simulink model "sensor_array_test"  (R2020a)
settings: Solver=VariableStepAuto  StartTime=0.0  StopTime=0.5  RelTol=1e-3
undefined symbols (not defined in the file or in its folder): duration, effort, index, joint_name, left_front, left_rear, model_name, right_front, right_rear, robotracer
libraries: robotgazebolib x24, simulink x3
settings Model: Creator=under  LastModifiedBy=under

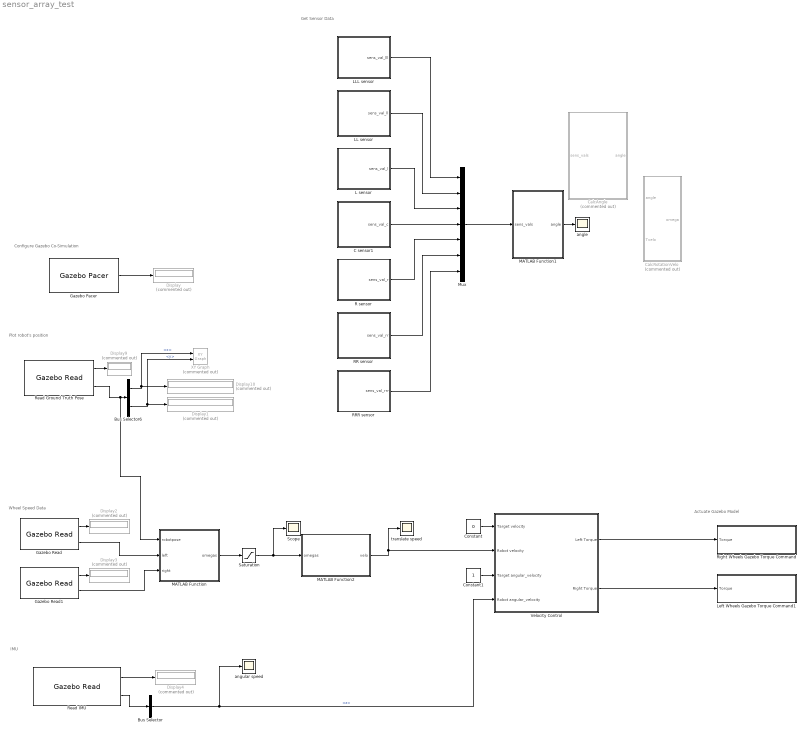
== system sensor_array_test ==
  note: Configure Gazebo Co-Simulation
  note: Plot robot's position
  note: Wheel Speed Data
  note: Actuate Gazebo Model
  note: IMU
  note: Get Sensor Data
  Bus Selector : BusSelector  OutputSignals=angular_velocity.z
  Bus Selector6 : BusSelector  OutputSignals=position.x,position.y
  C sensor1 : Subsystem
  CalcAngle : MATLAB Function  Commented=on  TreatAsAtomicUnit=on
  CalcRotationVelo : MATLAB Function  Commented=on  TreatAsAtomicUnit=on
  Constant : Constant  Value=0
  Constant1 : Constant
  Display{,1..4,9..10} (7 alike) : Display  Commented=on
  Gazebo Pacer : robotgazebolib/Gazebo Pacer  ResetBehavior=Reset Gazebo simulation time and scene  SampleTime=0.001
      settings: SourceProductBaseCode=RO
  Gazebo Read : robotgazebolib/Gazebo Read  topicSource=From Gazebo  topic=/gazebo/ground_truth/world_pose/robotracer/left_front_wheel  messageType=gazebo_msgs/Pose  sampleTime=0.001
      settings: SourceProductBaseCode=RO
  Gazebo Read1 : robotgazebolib/Gazebo Read  topicSource=From Gazebo  topic=/gazebo/ground_truth/world_pose/robotracer/right_front_wheel  messageType=gazebo_msgs/Pose  sampleTime=0.001
      settings: SourceProductBaseCode=RO
  L sensor : Subsystem
  LL sensor : Subsystem
  LLL sensor : Subsystem
  Left Wheels Gazebo Torque Command1 : Subsystem
  MATLAB Function : MATLAB Function  TreatAsAtomicUnit=on
  MATLAB Function1 : MATLAB Function  TreatAsAtomicUnit=on
  MATLAB Function2 : MATLAB Function  TreatAsAtomicUnit=on
  Mux : Mux  Inputs=7
  R sensor : Subsystem
  RR sensor : Subsystem
  RRR sensor : Subsystem
  Read Ground Truth Pose : robotgazebolib/Gazebo Read  topicSource=From Gazebo  topic=/gazebo/ground_truth/world_pose/robotracer/chassis  messageType=gazebo_msgs/Pose  sampleTime=0.001
      settings: SourceProductBaseCode=RO
  Read IMU : robotgazebolib/Gazebo Read  topicSource=From Gazebo  topic=/gazebo/default/robotracer/chassis/imu/imu  messageType=gazebo_msgs/IMU  sampleTime=0.01
      settings: SourceProductBaseCode=RO
  Right Wheels Gazebo Torque Command : Subsystem
  Saturation : Saturate  UpperLimit=90  LowerLimit=-90
  Scope : Scope
  Velocity Control : Subsystem
  XY Graph : simulink/Sinks/XY Graph  Commented=on  xmin=-1  xmax=1  ymin=-1  ymax=1  st=-1
  angle : Scope
  angular speed : Scope
  translate speed : Scope
  wires:
  Gazebo Pacer/1 -> Display/1
  Bus Selector6/1 -> XY Graph/1, Display10/1  "<x>"
  Bus Selector6/2 -> XY Graph/2, Display1/1  "<y>"
  MATLAB Function/1(omegas) -> Saturation/1
  Read Ground Truth Pose/2 -> MATLAB Function/1(robotpose), Bus Selector6/1
  Gazebo Read1/2 -> MATLAB Function/3(right)
  Gazebo Read/2 -> MATLAB Function/2(left)
  Gazebo Read1/1 -> Display3/1
  Gazebo Read/1 -> Display2/1
  Read Ground Truth Pose/1 -> Display9/1
  Saturation/1 -> MATLAB Function2/1(omegas), Scope/1
  MATLAB Function2/1(velo) -> Velocity Control/2(Robot velocity), translate speed/1
  Constant/1 -> Velocity Control/1(Target velocity)
  Read IMU/2 -> Bus Selector/1
  Read IMU/1 -> Display4/1
  Bus Selector/1 -> Velocity Control/4(Robot angular_velocity), angular speed/1  "<z>"
  Constant1/1 -> Velocity Control/3(Target angular_velocity)
  Velocity Control/1(Left Torque) -> Right Wheels Gazebo Torque Command/1(Torque)
  Velocity Control/2(Right Torque) -> Left Wheels Gazebo Torque Command1/1(Torque)
  C sensor1/1(sens_val_c) -> Mux/4
  L sensor/1(sens_val_l) -> Mux/3
  LL sensor/1(sens_val_ll) -> Mux/2
  LLL sensor/1(sens_val_lll) -> Mux/1
  R sensor/1(sens_val_r) -> Mux/5
  RR sensor/1(sens_val_rr) -> Mux/6
  RRR sensor/1(sens_val_rrr) -> Mux/7
  Mux/1 -> MATLAB Function1/1(sens_vals)
  MATLAB Function1/1(angle) -> angle/1

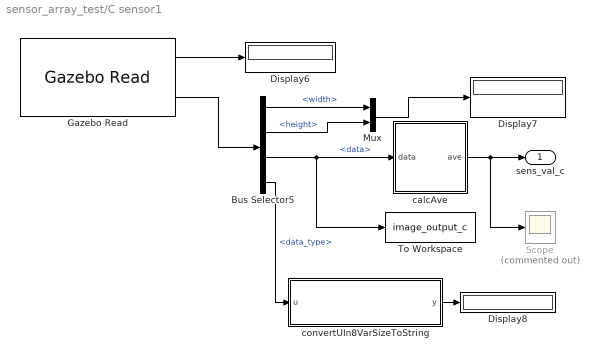
== system sensor_array_test/C sensor1 ==
  Bus Selector5 : BusSelector  OutputSignals=width,height,data,data_type
  Display6 : Display
  Display7 : Display
  Display8 : Display
  Gazebo Read : robotgazebolib/Gazebo Read  topicSource=From Gazebo  topic=/gazebo/default/robotracer/camera_link/camera_c/image  messageType=gazebo_msgs/Image  sampleTime=0.01
      settings: SourceProductBaseCode=RO
  Mux : Mux  Inputs=2
  Scope : Scope  Commented=on
  To Workspace : ToWorkspace  VariableName=image_output_c  SaveFormat=Structure With Time  SampleTime=-1
  calcAve : MATLAB Function  TreatAsAtomicUnit=on
  convertUIn8VarSizeToString : MATLAB Function  TreatAsAtomicUnit=on
  sens_val_c : Outport
  wires:
  calcAve/1(ave) -> sens_val_c/1, Scope/1
  Mux/1 -> Display7/1
  convertUIn8VarSizeToString/1(y) -> Display8/1
  Bus Selector5/2 -> Mux/2  "<height>"
  Bus Selector5/3 -> calcAve/1(data), To Workspace/1  "<data>"
  Bus Selector5/4 -> convertUIn8VarSizeToString/1(u)  "<data_type>"
  Gazebo Read/1 -> Display6/1
  Bus Selector5/1 -> Mux/1  "<width>"
  Gazebo Read/2 -> Bus Selector5/1

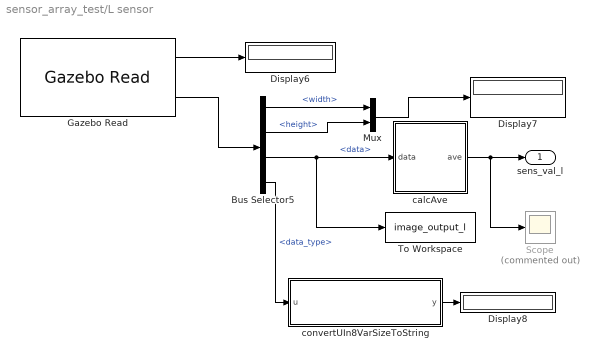
== system sensor_array_test/L sensor ==
  Bus Selector5 : BusSelector  OutputSignals=width,height,data,data_type
  Display6 : Display
  Display7 : Display
  Display8 : Display
  Gazebo Read : robotgazebolib/Gazebo Read  topicSource=From Gazebo  topic=/gazebo/default/robotracer/camera_link/camera_l/image  messageType=gazebo_msgs/Image  sampleTime=0.01
      settings: SourceProductBaseCode=RO
  Mux : Mux  Inputs=2
  Scope : Scope  Commented=on
  To Workspace : ToWorkspace  VariableName=image_output_l  SaveFormat=Structure With Time  SampleTime=-1
  calcAve : MATLAB Function  TreatAsAtomicUnit=on
  convertUIn8VarSizeToString : MATLAB Function  TreatAsAtomicUnit=on
  sens_val_l : Outport
  wires:
  calcAve/1(ave) -> sens_val_l/1, Scope/1
  Mux/1 -> Display7/1
  convertUIn8VarSizeToString/1(y) -> Display8/1
  Bus Selector5/2 -> Mux/2  "<height>"
  Bus Selector5/3 -> calcAve/1(data), To Workspace/1  "<data>"
  Bus Selector5/4 -> convertUIn8VarSizeToString/1(u)  "<data_type>"
  Gazebo Read/1 -> Display6/1
  Bus Selector5/1 -> Mux/1  "<width>"
  Gazebo Read/2 -> Bus Selector5/1

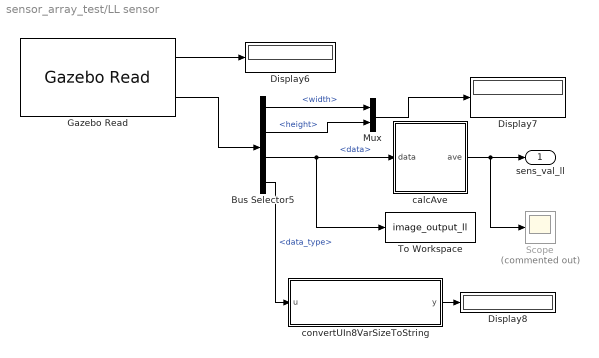
== system sensor_array_test/LL sensor ==
  Bus Selector5 : BusSelector  OutputSignals=width,height,data,data_type
  Display6 : Display
  Display7 : Display
  Display8 : Display
  Gazebo Read : robotgazebolib/Gazebo Read  topicSource=From Gazebo  topic=/gazebo/default/robotracer/camera_link/camera_ll/image  messageType=gazebo_msgs/Image  sampleTime=0.01
      settings: SourceProductBaseCode=RO
  Mux : Mux  Inputs=2
  Scope : Scope  Commented=on
  To Workspace : ToWorkspace  VariableName=image_output_ll  SaveFormat=Structure With Time  SampleTime=-1
  calcAve : MATLAB Function  TreatAsAtomicUnit=on
  convertUIn8VarSizeToString : MATLAB Function  TreatAsAtomicUnit=on
  sens_val_ll : Outport
  wires:
  calcAve/1(ave) -> sens_val_ll/1, Scope/1
  Mux/1 -> Display7/1
  convertUIn8VarSizeToString/1(y) -> Display8/1
  Bus Selector5/2 -> Mux/2  "<height>"
  Bus Selector5/3 -> calcAve/1(data), To Workspace/1  "<data>"
  Bus Selector5/4 -> convertUIn8VarSizeToString/1(u)  "<data_type>"
  Gazebo Read/1 -> Display6/1
  Bus Selector5/1 -> Mux/1  "<width>"
  Gazebo Read/2 -> Bus Selector5/1

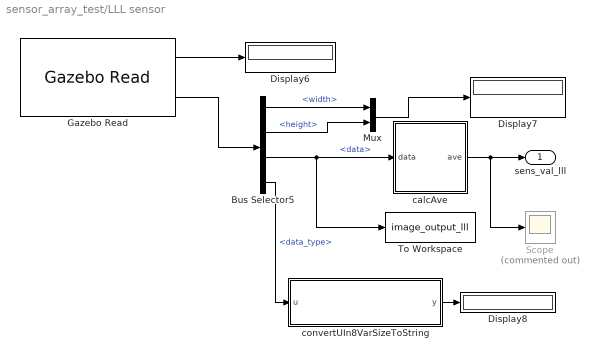
== system sensor_array_test/LLL sensor ==
  Bus Selector5 : BusSelector  OutputSignals=width,height,data,data_type
  Display6 : Display
  Display7 : Display
  Display8 : Display
  Gazebo Read : robotgazebolib/Gazebo Read  topicSource=From Gazebo  topic=/gazebo/default/robotracer/camera_link/camera_lll/image  messageType=gazebo_msgs/Image  sampleTime=0.01
      settings: SourceProductBaseCode=RO
  Mux : Mux  Inputs=2
  Scope : Scope  Commented=on
  To Workspace : ToWorkspace  VariableName=image_output_lll  SaveFormat=Structure With Time  SampleTime=-1
  calcAve : MATLAB Function  TreatAsAtomicUnit=on
  convertUIn8VarSizeToString : MATLAB Function  TreatAsAtomicUnit=on
  sens_val_lll : Outport
  wires:
  calcAve/1(ave) -> sens_val_lll/1, Scope/1
  Mux/1 -> Display7/1
  convertUIn8VarSizeToString/1(y) -> Display8/1
  Bus Selector5/2 -> Mux/2  "<height>"
  Bus Selector5/3 -> calcAve/1(data), To Workspace/1  "<data>"
  Bus Selector5/4 -> convertUIn8VarSizeToString/1(u)  "<data_type>"
  Gazebo Read/1 -> Display6/1
  Bus Selector5/1 -> Mux/1  "<width>"
  Gazebo Read/2 -> Bus Selector5/1

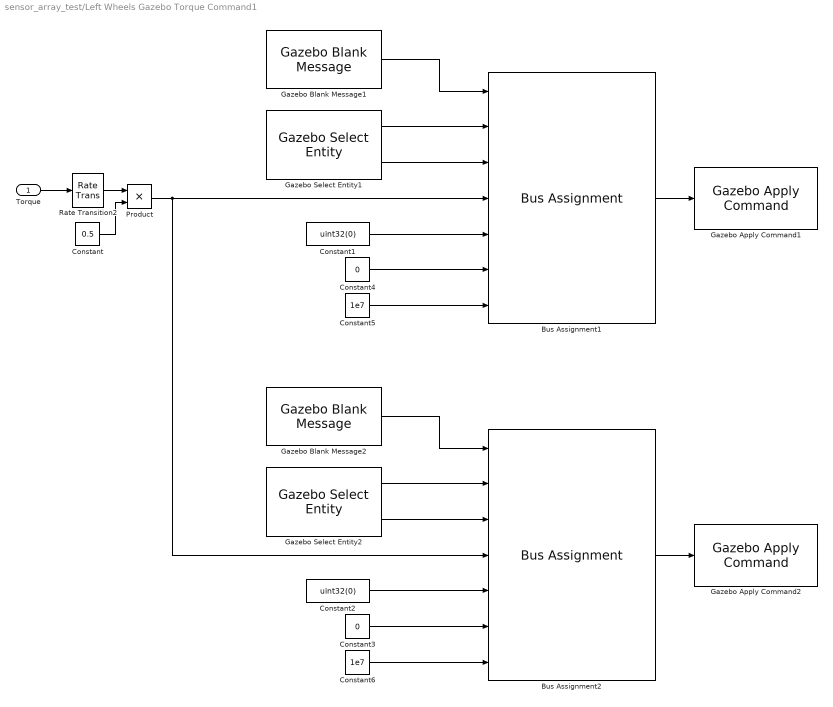
== system sensor_array_test/Left Wheels Gazebo Torque Command1 ==
  Torque : Inport
  Bus Assignment1 : BusAssignment  AssignedSignals=model_name,joint_name,effort,index,duration.seconds,duration.nano_seconds
  Bus Assignment2 : BusAssignment  AssignedSignals=model_name,joint_name,effort,index,duration.seconds,duration.nano_seconds
  Constant : Constant  Value=0.5
  Constant1 : Constant  Value=uint32(0)
  Constant2 : Constant  Value=uint32(0)
  Constant3 : Constant  Value=0
  Constant4 : Constant  Value=0
  Constant5 : Constant  Value=1e7
  Constant6 : Constant  Value=1e7
  Gazebo Apply Command1 : robotgazebolib/Gazebo Apply Command  cmdType=ApplyJointTorque  sampleTime=0.01
      settings: SourceProductBaseCode=RO
  Gazebo Apply Command2 : robotgazebolib/Gazebo Apply Command  cmdType=ApplyJointTorque  sampleTime=0.01
      settings: SourceProductBaseCode=RO
  Gazebo Blank Message1 : robotgazebolib/Gazebo Blank Message  msgType=ApplyJointTorque  sampleTime=0.01  busName='Gazebo_SL_Bus_gazebo_msgs_ApplyJointTorque'
      settings: SourceProductBaseCode=RO
  Gazebo Blank Message2 : robotgazebolib/Gazebo Blank Message  msgType=ApplyJointTorque  sampleTime=0.01  busName='Gazebo_SL_Bus_gazebo_msgs_ApplyJointTorque'
      settings: SourceProductBaseCode=RO
  Gazebo Select Entity1 : robotgazebolib/Gazebo Select Entity  modelElemName=robotracer/left_front  outputArraySize=128  OutputLabel=Joint  SelectType=Joint
      settings: SourceProductBaseCode=RO
  Gazebo Select Entity2 : robotgazebolib/Gazebo Select Entity  modelElemName=robotracer/left_rear  outputArraySize=128  OutputLabel=Joint  SelectType=Joint
      settings: SourceProductBaseCode=RO
  Product : Product
  Rate Transition2 : RateTransition
  wires:
  Bus Assignment1/1 -> Gazebo Apply Command1/1
  Constant5/1 -> Bus Assignment1/7
  Gazebo Blank Message1/1 -> Bus Assignment1/1
  Gazebo Select Entity1/2 -> Bus Assignment1/3
  Gazebo Select Entity1/1 -> Bus Assignment1/2
  Constant4/1 -> Bus Assignment1/6
  Constant1/1 -> Bus Assignment1/5
  Gazebo Select Entity2/1 -> Bus Assignment2/2
  Constant6/1 -> Bus Assignment2/7
  Constant2/1 -> Bus Assignment2/5
  Constant3/1 -> Bus Assignment2/6
  Gazebo Select Entity2/2 -> Bus Assignment2/3
  Torque/1 -> Rate Transition2/1
  Gazebo Blank Message2/1 -> Bus Assignment2/1
  Bus Assignment2/1 -> Gazebo Apply Command2/1
  Constant/1 -> Product/2
  Rate Transition2/1 -> Product/1
  Product/1 -> Bus Assignment2/4, Bus Assignment1/4

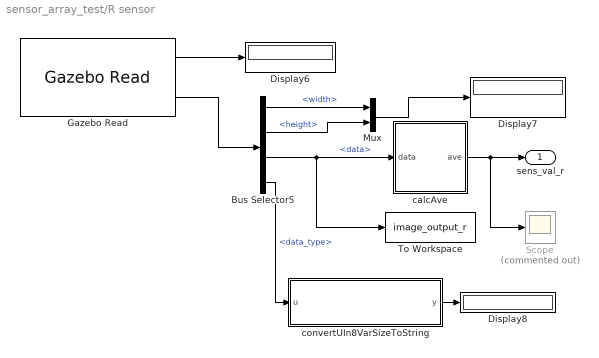
== system sensor_array_test/R sensor ==
  Bus Selector5 : BusSelector  OutputSignals=width,height,data,data_type
  Display6 : Display
  Display7 : Display
  Display8 : Display
  Gazebo Read : robotgazebolib/Gazebo Read  topicSource=From Gazebo  topic=/gazebo/default/robotracer/camera_link/camera_r/image  messageType=gazebo_msgs/Image  sampleTime=0.01
      settings: SourceProductBaseCode=RO
  Mux : Mux  Inputs=2
  Scope : Scope  Commented=on
  To Workspace : ToWorkspace  VariableName=image_output_r  SaveFormat=Structure With Time  SampleTime=-1
  calcAve : MATLAB Function  TreatAsAtomicUnit=on
  convertUIn8VarSizeToString : MATLAB Function  TreatAsAtomicUnit=on
  sens_val_r : Outport
  wires:
  calcAve/1(ave) -> sens_val_r/1, Scope/1
  Mux/1 -> Display7/1
  convertUIn8VarSizeToString/1(y) -> Display8/1
  Bus Selector5/2 -> Mux/2  "<height>"
  Bus Selector5/3 -> calcAve/1(data), To Workspace/1  "<data>"
  Bus Selector5/4 -> convertUIn8VarSizeToString/1(u)  "<data_type>"
  Gazebo Read/1 -> Display6/1
  Bus Selector5/1 -> Mux/1  "<width>"
  Gazebo Read/2 -> Bus Selector5/1

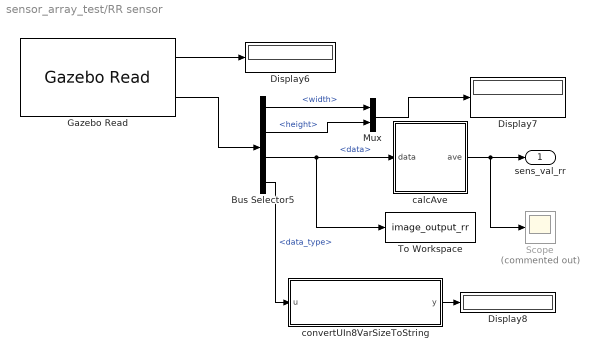
== system sensor_array_test/RR sensor ==
  Bus Selector5 : BusSelector  OutputSignals=width,height,data,data_type
  Display6 : Display
  Display7 : Display
  Display8 : Display
  Gazebo Read : robotgazebolib/Gazebo Read  topicSource=From Gazebo  topic=/gazebo/default/robotracer/camera_link/camera_rr/image  messageType=gazebo_msgs/Image  sampleTime=0.01
      settings: SourceProductBaseCode=RO
  Mux : Mux  Inputs=2
  Scope : Scope  Commented=on
  To Workspace : ToWorkspace  VariableName=image_output_rr  SaveFormat=Structure With Time  SampleTime=-1
  calcAve : MATLAB Function  TreatAsAtomicUnit=on
  convertUIn8VarSizeToString : MATLAB Function  TreatAsAtomicUnit=on
  sens_val_rr : Outport
  wires:
  calcAve/1(ave) -> sens_val_rr/1, Scope/1
  Mux/1 -> Display7/1
  convertUIn8VarSizeToString/1(y) -> Display8/1
  Bus Selector5/2 -> Mux/2  "<height>"
  Bus Selector5/3 -> calcAve/1(data), To Workspace/1  "<data>"
  Bus Selector5/4 -> convertUIn8VarSizeToString/1(u)  "<data_type>"
  Gazebo Read/1 -> Display6/1
  Bus Selector5/1 -> Mux/1  "<width>"
  Gazebo Read/2 -> Bus Selector5/1

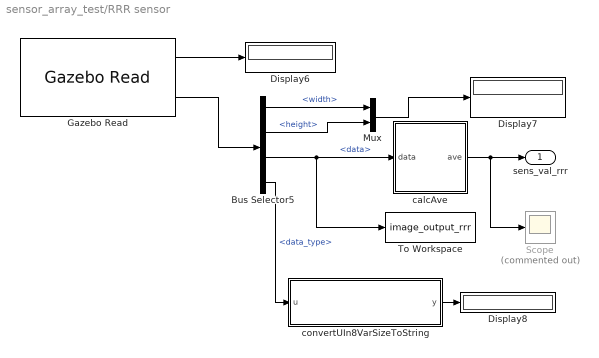
== system sensor_array_test/RRR sensor ==
  Bus Selector5 : BusSelector  OutputSignals=width,height,data,data_type
  Display6 : Display
  Display7 : Display
  Display8 : Display
  Gazebo Read : robotgazebolib/Gazebo Read  topicSource=From Gazebo  topic=/gazebo/default/robotracer/camera_link/camera_rrr/image  messageType=gazebo_msgs/Image  sampleTime=0.01
      settings: SourceProductBaseCode=RO
  Mux : Mux  Inputs=2
  Scope : Scope  Commented=on
  To Workspace : ToWorkspace  VariableName=image_output_rrr  SaveFormat=Structure With Time  SampleTime=-1
  calcAve : MATLAB Function  TreatAsAtomicUnit=on
  convertUIn8VarSizeToString : MATLAB Function  TreatAsAtomicUnit=on
  sens_val_rrr : Outport
  wires:
  calcAve/1(ave) -> sens_val_rrr/1, Scope/1
  Mux/1 -> Display7/1
  convertUIn8VarSizeToString/1(y) -> Display8/1
  Bus Selector5/2 -> Mux/2  "<height>"
  Bus Selector5/3 -> calcAve/1(data), To Workspace/1  "<data>"
  Bus Selector5/4 -> convertUIn8VarSizeToString/1(u)  "<data_type>"
  Gazebo Read/1 -> Display6/1
  Bus Selector5/1 -> Mux/1  "<width>"
  Gazebo Read/2 -> Bus Selector5/1

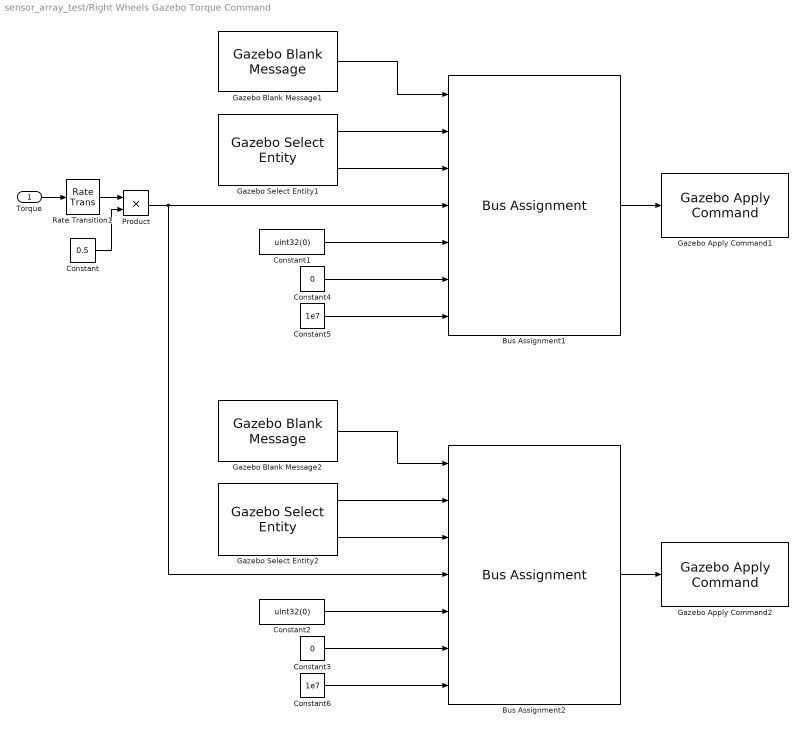
== system sensor_array_test/Right Wheels Gazebo Torque Command ==
  Torque : Inport
  Bus Assignment1 : BusAssignment  AssignedSignals=model_name,joint_name,effort,index,duration.seconds,duration.nano_seconds
  Bus Assignment2 : BusAssignment  AssignedSignals=model_name,joint_name,effort,index,duration.seconds,duration.nano_seconds
  Constant : Constant  Value=0.5
  Constant1 : Constant  Value=uint32(0)
  Constant2 : Constant  Value=uint32(0)
  Constant3 : Constant  Value=0
  Constant4 : Constant  Value=0
  Constant5 : Constant  Value=1e7
  Constant6 : Constant  Value=1e7
  Gazebo Apply Command1 : robotgazebolib/Gazebo Apply Command  cmdType=ApplyJointTorque  sampleTime=0.001
      settings: SourceProductBaseCode=RO
  Gazebo Apply Command2 : robotgazebolib/Gazebo Apply Command  cmdType=ApplyJointTorque  sampleTime=0.001
      settings: SourceProductBaseCode=RO
  Gazebo Blank Message1 : robotgazebolib/Gazebo Blank Message  msgType=ApplyJointTorque  sampleTime=0.001  busName='Gazebo_SL_Bus_gazebo_msgs_ApplyJointTorque'
      settings: SourceProductBaseCode=RO
  Gazebo Blank Message2 : robotgazebolib/Gazebo Blank Message  msgType=ApplyJointTorque  sampleTime=0.001  busName='Gazebo_SL_Bus_gazebo_msgs_ApplyJointTorque'
      settings: SourceProductBaseCode=RO
  Gazebo Select Entity1 : robotgazebolib/Gazebo Select Entity  modelElemName=robotracer/right_front  outputArraySize=128  OutputLabel=Joint  SelectType=Joint
      settings: SourceProductBaseCode=RO
  Gazebo Select Entity2 : robotgazebolib/Gazebo Select Entity  modelElemName=robotracer/right_rear  outputArraySize=128  OutputLabel=Joint  SelectType=Joint
      settings: SourceProductBaseCode=RO
  Product : Product
  Rate Transition1 : RateTransition
  wires:
  Bus Assignment1/1 -> Gazebo Apply Command1/1
  Constant5/1 -> Bus Assignment1/7
  Gazebo Blank Message1/1 -> Bus Assignment1/1
  Gazebo Select Entity1/2 -> Bus Assignment1/3
  Gazebo Select Entity1/1 -> Bus Assignment1/2
  Constant4/1 -> Bus Assignment1/6
  Rate Transition1/1 -> Product/1
  Constant1/1 -> Bus Assignment1/5
  Gazebo Select Entity2/1 -> Bus Assignment2/2
  Constant6/1 -> Bus Assignment2/7
  Constant2/1 -> Bus Assignment2/5
  Constant3/1 -> Bus Assignment2/6
  Gazebo Select Entity2/2 -> Bus Assignment2/3
  Torque/1 -> Rate Transition1/1
  Gazebo Blank Message2/1 -> Bus Assignment2/1
  Bus Assignment2/1 -> Gazebo Apply Command2/1
  Constant/1 -> Product/2
  Product/1 -> Bus Assignment1/4, Bus Assignment2/4

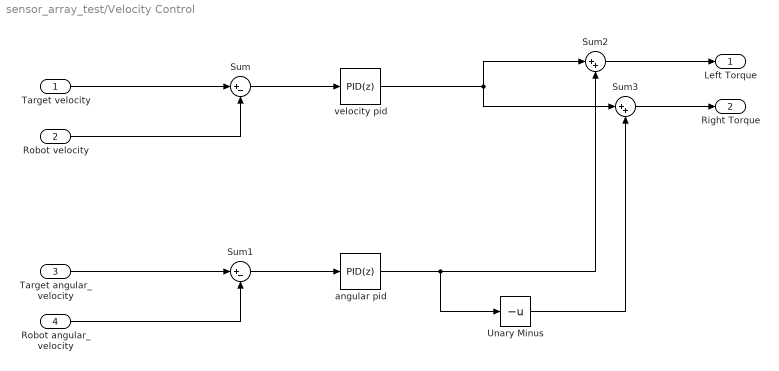
== system sensor_array_test/Velocity Control ==
  Target velocity : Inport
  Robot velocity : Inport  Port=2
  Target angular_velocity : Inport  Port=3
  Robot angular_velocity : Inport  Port=4
  Sum : Sum  Inputs=|+-
  Sum1 : Sum  Inputs=|+-
  Sum2 : Sum  Inputs=|++
  Sum3 : Sum  Inputs=|++
  Unary Minus : UnaryMinus
  angular pid : simulink/Continuous/PID Controller  Controller=PID  Form=Parallel  TimeDomain=Discrete-time  UseExternalTs=off  SampleTime=-1  IntegratorMethod=Forward Euler  FilterMethod=Forward Euler  ControllerParametersSource=internal  P=0.00035878  I=0.0049875  D=0  UseFilter=on  N=100  TunerSelectOption=Transfer Function Based (PID Tuner App)  InitialConditionSource=internal  InitialConditionForIntegrator=0  InitialConditionForFilter=0  DifferentiatorICPrevScaledInput=0  ExternalReset=none  TrackingMode=off  Kt=1  LimitOutput=off  UpperSaturationLimit=inf  LowerSaturationLimit=-inf  LinearizeAsGain=off  AntiWindupMode=none  Kb=1  POutMin=[]  POutMax=[]  IOutMin=[]  IOutMax=[]  DOutMin=[]  DOutMax=[]  NOutMin=[]  NOutMax=[]  SumOutMin=[]  SumOutMax=[]  SaturationOutMin=[]  SaturationOutMax=[]  PParamMin=[]  PParamMax=[]  IParamMin=[]  IParamMax=[]  DParamMin=[]  DParamMax=[]  NParamMin=[]  NParamMax=[]  KbParamMin=[]  KbParamMax=[]  KtParamMin=[]  KtParamMax=[]  KbOutMin=[]  KbOutMax=[]  KtOutMin=[]  KtOutMax=[]  IntegratorOutMin=[]  IntegratorOutMax=[]  FilterOutMin=[]  FilterOutMax=[]  SumI1OutMin=[]  SumI1OutMax=[]  SumI2OutMin=[]  SumI2OutMax=[]  SumI3OutMin=[]  SumI3OutMax=[]  SumI4OutMin=[]  SumI4OutMax=[]  SumDOutMin=[]  SumDOutMax=[]  DifferentiatorOutMin=[]  DifferentiatorOutMax=[]  FilterDiffOutCoefMin=[]  FilterDiffOutCoefMax=[]  ReciprocalOutMin=[]  ReciprocalOutMax=[]  SumDenOutMin=[]  SumDenOutMax=[]  SumNumOutMin=[]  SumNumOutMax=[]  DivideOutMin=[]  DivideOutMax=[]  UdiffTsProdOutMin=[]  UdiffTsProdOutMax=[]  NTsProdOutMin=[]  NTsProdOutMax=[]  UintegralTsProdOutMin=[]  UintegralTsProdOutMax=[]  UngainTsProdOutMin=[]  UngainTsProdOutMax=[]  IntegratorContinuousStateAttributes=''  IntegratorStateMustResolveToSignalObject=off  IntegratorRTWStateStorageClass=Auto  FilterContinuousStateAttributes=''  FilterStateMustResolveToSignalObject=off  FilterRTWStateStorageClass=Auto  ParallelPVariant=InternalParameters  IdealPVariant=Disabled  IVariant=InternalParameters  DVariant=InternalParameters  IntegratorVariant=Discrete  SatVariant=Disabled  AWVariant=Passthrough  PCopyVariant=Disabled  TRVariant=Disabled  FdbkBlocksVariant=Forward  IdealPFdbkVariant=Disabled  SatFdbkVariant=Disabled  DerivativeFilterVariant=ForwardEulerFilter  NVariant=InternalParameters  NCopyVariant=Disabled  FilterICVariant=InternalICsFilter  IntegratorICVariant=InternalICs  ExternalResetVariant=Disabled  TRSumVariant=Passthrough  SumFdbkVariant=Disabled  SumVariant=Sum_PID  TsampFilterVariant=InternalTs  TsampNgainVariant=Passthrough  TsampIntegralVariant=Passthrough
  velocity pid : simulink/Continuous/PID Controller  Controller=PID  Form=Parallel  TimeDomain=Discrete-time  UseExternalTs=off  SampleTime=-1  IntegratorMethod=Forward Euler  FilterMethod=Forward Euler  ControllerParametersSource=internal  P=0.0011697  I=0.0046226  D=0  UseFilter=on  N=100  TunerSelectOption=Transfer Function Based (PID Tuner App)  InitialConditionSource=internal  InitialConditionForIntegrator=0  InitialConditionForFilter=0  DifferentiatorICPrevScaledInput=0  ExternalReset=none  TrackingMode=off  Kt=1  LimitOutput=off  UpperSaturationLimit=inf  LowerSaturationLimit=-inf  LinearizeAsGain=off  AntiWindupMode=none  Kb=1  POutMin=[]  POutMax=[]  IOutMin=[]  IOutMax=[]  DOutMin=[]  DOutMax=[]  NOutMin=[]  NOutMax=[]  SumOutMin=[]  SumOutMax=[]  SaturationOutMin=[]  SaturationOutMax=[]  PParamMin=[]  PParamMax=[]  IParamMin=[]  IParamMax=[]  DParamMin=[]  DParamMax=[]  NParamMin=[]  NParamMax=[]  KbParamMin=[]  KbParamMax=[]  KtParamMin=[]  KtParamMax=[]  KbOutMin=[]  KbOutMax=[]  KtOutMin=[]  KtOutMax=[]  IntegratorOutMin=[]  IntegratorOutMax=[]  FilterOutMin=[]  FilterOutMax=[]  SumI1OutMin=[]  SumI1OutMax=[]  SumI2OutMin=[]  SumI2OutMax=[]  SumI3OutMin=[]  SumI3OutMax=[]  SumI4OutMin=[]  SumI4OutMax=[]  SumDOutMin=[]  SumDOutMax=[]  DifferentiatorOutMin=[]  DifferentiatorOutMax=[]  FilterDiffOutCoefMin=[]  FilterDiffOutCoefMax=[]  ReciprocalOutMin=[]  ReciprocalOutMax=[]  SumDenOutMin=[]  SumDenOutMax=[]  SumNumOutMin=[]  SumNumOutMax=[]  DivideOutMin=[]  DivideOutMax=[]  UdiffTsProdOutMin=[]  UdiffTsProdOutMax=[]  NTsProdOutMin=[]  NTsProdOutMax=[]  UintegralTsProdOutMin=[]  UintegralTsProdOutMax=[]  UngainTsProdOutMin=[]  UngainTsProdOutMax=[]  IntegratorContinuousStateAttributes=''  IntegratorStateMustResolveToSignalObject=off  IntegratorRTWStateStorageClass=Auto  FilterContinuousStateAttributes=''  FilterStateMustResolveToSignalObject=off  FilterRTWStateStorageClass=Auto  ParallelPVariant=InternalParameters  IdealPVariant=Disabled  IVariant=InternalParameters  DVariant=InternalParameters  IntegratorVariant=Discrete  SatVariant=Disabled  AWVariant=Passthrough  PCopyVariant=Disabled  TRVariant=Disabled  FdbkBlocksVariant=Forward  IdealPFdbkVariant=Disabled  SatFdbkVariant=Disabled  DerivativeFilterVariant=ForwardEulerFilter  NVariant=InternalParameters  NCopyVariant=Disabled  FilterICVariant=InternalICsFilter  IntegratorICVariant=InternalICs  ExternalResetVariant=Disabled  TRSumVariant=Passthrough  SumFdbkVariant=Disabled  SumVariant=Sum_PID  TsampFilterVariant=InternalTs  TsampNgainVariant=Passthrough  TsampIntegralVariant=Passthrough
  Left Torque : Outport
  Right Torque : Outport  Port=2
  wires:
  Target velocity/1 -> Sum/1
  Sum/1 -> velocity pid/1
  velocity pid/1 -> Sum3/1, Sum2/1
  Robot velocity/1 -> Sum/2
  Unary Minus/1 -> Sum3/2
  Target angular_velocity/1 -> Sum1/1
  Sum1/1 -> angular pid/1
  angular pid/1 -> Sum2/2, Unary Minus/1
  Robot angular_velocity/1 -> Sum1/2
  Sum2/1 -> Left Torque/1
  Sum3/1 -> Right Torque/1

== matlab function sensor_array_test/RR sensor/convertUIn8VarSizeToString ==
  data: u input; y output string
function y = convertUInt8VarSizeToString(u)

y = convertCharsToStrings(char(u'));

== matlab function sensor_array_test/MATLAB Function ==
  data: robotpose input; omegas output; left input; right input
function omegas = computeWheelVelocities(robotpose, left, right)
%computeWheelVelocities computes wheel velocity based on rate of change of
%the yaw angle of the wheel relative to its original mount on the robot
%body

persistent initAngles
if isempty(initAngles)
    initAngles = zeros(2, 1);
end
sampleTime = 0.001;

% compute rotation between wheel original mount on the robot body and world
% frame
robotRtom = quat2rotm([robotpose.orientation.w, robotpose.orientation.x, robotpose.orientation.y, robotpose.orientation.z]);
originalWheelMount = robotRtom * eul2rotm([pi/2 pi/2 0]);

% get rotation between wheel and the world frame
leftRtom = quat2rotm([left.orientation.w, left.orientation.x, left.orientation.y, left.orientation.z]);
rightRtom = quat2rotm([right.orientation.w, right.orientation.x, right.orientation.y, right.orientation.z]);

% compute relative rotation between wheel and its original mount
leftRotation = rotm2eul(originalWheelMount' * leftRtom);
rightRotation = rotm2eul(originalWheelMount' * rightRtom);

% compute angluar velocity using the angle difference between the current
% angle pose and the the angle pose in last time step
angles = [leftRotation(1); rightRotation(1)];
omegas = angdiff(initAngles, angles) / sampleTime;
if omegas(1, 1) < -1000
    omegas(1, 1) = 0;
end
if omegas(2, 1) < -1000
    omegas(2, 1) = 0;
end
initAngles = angles;

== matlab function sensor_array_test/R sensor/calcAve ==
  data: data input; ave output
function ave = calcAve(data)    
    if length(data) >= 3
        width = 10;
        height = 10;
        numOutputChannels = 3;
        indexBase = (1:numOutputChannels:width*height*numOutputChannels)';
        index = zeros(numel(indexBase),numOutputChannels);
        for i = 1:numOutputChannels
            % Construct it as column-major index to ease later reshape
            index(:, i) = indexBase + i - 1;
        end

        % Reshape the data into a width x height x numOutputChannels matrix
        img = reshape(data(index), width, height, numOutputChannels);

        % Since reshape works column-wise, bring image back to
        % row-major order (transpose of 1st and 2nd dimension
        % Result will be a height x width x numOutputChannels image matrix
        img = permute(img, [2 1 3]);

        ave = mean(img(:, :, 1), 'all');
        
        % デバッグ用
        %{
        disp('data: ')
        disp(data(1))

        disp('mean: ')
        disp(mean(data))

        disp('len: ')
        disp(length(data))
    
        disp('R datas: ')
        disp(img(:, :, 1))
        
        disp('R mean: ')
        disp(ave)
        %}
    else
        ave = 0;
        
    end
        
end

== matlab function sensor_array_test/R sensor/convertUIn8VarSizeToString ==
  data: u input; y output string
function y = convertUInt8VarSizeToString(u)

y = convertCharsToStrings(char(u'));

== matlab function sensor_array_test/CalcAngle ==
  data: sens_vals input size=[1. 20]; angle output; SensorAngle_ data_store_memory; SensorNumber_ data_store_memory
function angle = fcn(sens_vals)

    sensor_num = 7;
    angle = 120;
    
    disp(sens_vals)
    
%     AngleBetweenSensor = deg2rad(SensorAngle_ / SensorNumber_); %[rad]
%     AllSensorNumer = SensorNumber_ * 2 + 1;
%     CenterNumber = ceil(AllSensorNumer / 2); %Number of center sensor
% 
%     [~, Index] = max(sens_vals);
%     
%     if Index == 1
%         NormAD = [0, sens_vals(1, Index) / sens_vals(1, Index), sens_vals(1, Index + 1) / sens_vals(1, Index)];
%     elseif Index == AllSensorNumer
%         NormAD = [sens_vals(1, Index - 1) / sens_vals(1, Index), sens_vals(1, Index) / sens_vals(1, Index), 0];
%     else
%         NormAD = [sens_vals(1, Index - 1) / sens_vals(1, Index), sens_vals(1, Index) / sens_vals(1, Index), sens_vals(1, Index + 1) / sens_vals(1, Index)];
%     end
%     
%     ratio = NormAD(1) -  NormAD(3);
%     StandardAngle = (CenterNumber - Index(1, 1)) * AngleBetweenSensor;
%     DeltaTheta = (AngleBetweenSensor / 2)  * ratio;
%     
%     
%     angle = StandardAngle + DeltaTheta;
    angle = 0;

end

== matlab function sensor_array_test/CalcRotationVelo ==
  settings: updateMethod=DISCRETE
  data: angle input; omega output; L_ data_store_memory; Tvelo input
function omega = fcn(angle, Tvelo)
    global L_
    
    if angle ~= 0
        Radius = L_ / tan(angle);
    else
        Radius = 9e10;
        
    end
    
    omega = -Tvelo / (Radius * 1e-3);    
end

== matlab function sensor_array_test/MATLAB Function1 ==
  data: sens_vals input; angle output
function angle = calcAngle(sens_vals) % sens_valsは行方向に格納される
    disp(sens_vals(:, :));
    
    sensor_num = 7; % 奇数
    angle = deg2rad(120); % deg
    angle_step = (angle / 2) / ((sensor_num - 1) / 2); % rad
%     half_thetas = 0 : angle_step : angle / 2;

%     reverse_thetas = -flip(half_thetas);
%     reverse_thetas(end) = [];
%     ref_thetas = [reverse_thetas, half_thetas];
    
    center_num = ceil(sensor_num / 2); %Number of center sensor
    
    [~, index] = max(sens_vals);
    
    if index == 1
        NormAD = [0, sens_vals(index, :) / sens_vals(index, :), sens_vals(index + 1, :) / sens_vals(index, :)];
    elseif index == sensor_num
        NormAD = [sens_vals(index - 1, :) / sens_vals(index, :), sens_vals(index, :) / sens_vals(index, :), 0];
    else
        NormAD = [sens_vals(index - 1, :) / sens_vals(index, :), sens_vals(index, :) / sens_vals(index, :), sens_vals(index + 1, :) / sens_vals(index, :)];
    end

    ratio = NormAD(1) -  NormAD(3);
    StandardAngle = (center_num - index(1, 1)) * angle_step;
    DeltaTheta = (angle_step / 2)  * ratio;
    
    angle = StandardAngle + DeltaTheta;
end

== matlab function sensor_array_test/LL sensor/calcAve ==
  data: data input; ave output
function ave = calcAve(data)    
    if length(data) >= 3
        width = 10;
        height = 10;
        numOutputChannels = 3;
        indexBase = (1:numOutputChannels:width*height*numOutputChannels)';
        index = zeros(numel(indexBase),numOutputChannels);
        for i = 1:numOutputChannels
            % Construct it as column-major index to ease later reshape
            index(:, i) = indexBase + i - 1;
        end

        % Reshape the data into a width x height x numOutputChannels matrix
        img = reshape(data(index), width, height, numOutputChannels);

        % Since reshape works column-wise, bring image back to
        % row-major order (transpose of 1st and 2nd dimension
        % Result will be a height x width x numOutputChannels image matrix
        img = permute(img, [2 1 3]);

        ave = mean(img(:, :, 1), 'all');
        
        % デバッグ用
        %{
        disp('data: ')
        disp(data(1))

        disp('mean: ')
        disp(mean(data))

        disp('len: ')
        disp(length(data))
    
        disp('R datas: ')
        disp(img(:, :, 1))
        
        disp('R mean: ')
        disp(ave)
        %}
    else
        ave = 0;
        
    end
        
end

== matlab function sensor_array_test/MATLAB Function2 ==
  data: omegas input; velo output
function velo = omegas2velocity(omegas)
    wheel_radius = 0.010; %[m]
    m_per_omega = 2 * pi * wheel_radius;
    
    velo = mean(omegas, 'all') * m_per_omega;

== matlab function sensor_array_test/LL sensor/convertUIn8VarSizeToString ==
  data: u input; y output string
function y = convertUInt8VarSizeToString(u)

y = convertCharsToStrings(char(u'));

== matlab function sensor_array_test/LLL sensor/calcAve ==
  data: data input; ave output
function ave = calcAve(data)    
    if length(data) >= 3
        width = 10;
        height = 10;
        numOutputChannels = 3;
        indexBase = (1:numOutputChannels:width*height*numOutputChannels)';
        index = zeros(numel(indexBase),numOutputChannels);
        for i = 1:numOutputChannels
            % Construct it as column-major index to ease later reshape
            index(:, i) = indexBase + i - 1;
        end

        % Reshape the data into a width x height x numOutputChannels matrix
        img = reshape(data(index), width, height, numOutputChannels);

        % Since reshape works column-wise, bring image back to
        % row-major order (transpose of 1st and 2nd dimension
        % Result will be a height x width x numOutputChannels image matrix
        img = permute(img, [2 1 3]);

        ave = mean(img(:, :, 1), 'all');
        
        % デバッグ用
        %{
        disp('data: ')
        disp(data(1))

        disp('mean: ')
        disp(mean(data))

        disp('len: ')
        disp(length(data))
    
        disp('R datas: ')
        disp(img(:, :, 1))
        
        disp('R mean: ')
        disp(ave)
        %}
    else
        ave = 0;
        
    end
        
end

== matlab function sensor_array_test/LLL sensor/convertUIn8VarSizeToString ==
  data: u input; y output string
function y = convertUInt8VarSizeToString(u)

y = convertCharsToStrings(char(u'));

== matlab function sensor_array_test/C sensor1/calcAve ==
  data: data input; ave output
function ave = calcAve(data)    
    if length(data) >= 3
        width = 10;
        height = 10;
        numOutputChannels = 3;
        indexBase = (1:numOutputChannels:width*height*numOutputChannels)';
        index = zeros(numel(indexBase),numOutputChannels);
        for i = 1:numOutputChannels
            % Construct it as column-major index to ease later reshape
            index(:, i) = indexBase + i - 1;
        end

        % Reshape the data into a width x height x numOutputChannels matrix
        img = reshape(data(index), width, height, numOutputChannels);

        % Since reshape works column-wise, bring image back to
        % row-major order (transpose of 1st and 2nd dimension
        % Result will be a height x width x numOutputChannels image matrix
        img = permute(img, [2 1 3]);

        ave = mean(img(:, :, 1), 'all');
        
        % デバッグ用
        %{
        disp('data: ')
        disp(data(1))

        disp('mean: ')
        disp(mean(data))

        disp('len: ')
        disp(length(data))
    
        disp('R datas: ')
        disp(img(:, :, 1))
        
        disp('R mean: ')
        disp(ave)
        %}
    else
        ave = 0;
        
    end
        
end

== matlab function sensor_array_test/C sensor1/convertUIn8VarSizeToString ==
  data: u input; y output string
function y = convertUInt8VarSizeToString(u)

y = convertCharsToStrings(char(u'));

== matlab function sensor_array_test/L sensor/calcAve ==
  data: data input; ave output
function ave = calcAve(data)    
    if length(data) >= 3
        width = 10;
        height = 10;
        numOutputChannels = 3;
        indexBase = (1:numOutputChannels:width*height*numOutputChannels)';
        index = zeros(numel(indexBase),numOutputChannels);
        for i = 1:numOutputChannels
            % Construct it as column-major index to ease later reshape
            index(:, i) = indexBase + i - 1;
        end

        % Reshape the data into a width x height x numOutputChannels matrix
        img = reshape(data(index), width, height, numOutputChannels);

        % Since reshape works column-wise, bring image back to
        % row-major order (transpose of 1st and 2nd dimension
        % Result will be a height x width x numOutputChannels image matrix
        img = permute(img, [2 1 3]);

        ave = mean(img(:, :, 1), 'all');
        
        % デバッグ用
        %{
        disp('data: ')
        disp(data(1))

        disp('mean: ')
        disp(mean(data))

        disp('len: ')
        disp(length(data))
    
        disp('R datas: ')
        disp(img(:, :, 1))
        
        disp('R mean: ')
        disp(ave)
        %}
    else
        ave = 0;
        
    end
        
end

== matlab function sensor_array_test/L sensor/convertUIn8VarSizeToString ==
  data: u input; y output string
function y = convertUInt8VarSizeToString(u)

y = convertCharsToStrings(char(u'));

== matlab function sensor_array_test/RRR sensor/calcAve ==
  data: data input; ave output
function ave = calcAve(data)    
    if length(data) >= 3
        width = 10;
        height = 10;
        numOutputChannels = 3;
        indexBase = (1:numOutputChannels:width*height*numOutputChannels)';
        index = zeros(numel(indexBase),numOutputChannels);
        for i = 1:numOutputChannels
            % Construct it as column-major index to ease later reshape
            index(:, i) = indexBase + i - 1;
        end

        % Reshape the data into a width x height x numOutputChannels matrix
        img = reshape(data(index), width, height, numOutputChannels);

        % Since reshape works column-wise, bring image back to
        % row-major order (transpose of 1st and 2nd dimension
        % Result will be a height x width x numOutputChannels image matrix
        img = permute(img, [2 1 3]);

        ave = mean(img(:, :, 1), 'all');
        
        % デバッグ用
        %{
        disp('data: ')
        disp(data(1))

        disp('mean: ')
        disp(mean(data))

        disp('len: ')
        disp(length(data))
    
        disp('R datas: ')
        disp(img(:, :, 1))
        
        disp('R mean: ')
        disp(ave)
        %}
    else
        ave = 0;
        
    end
        
end

== matlab function sensor_array_test/RRR sensor/convertUIn8VarSizeToString ==
  data: u input; y output string
function y = convertUInt8VarSizeToString(u)

y = convertCharsToStrings(char(u'));

== matlab function sensor_array_test/RR sensor/calcAve ==
  data: data input; ave output
function ave = calcAve(data)    
    if length(data) >= 3
        width = 10;
        height = 10;
        numOutputChannels = 3;
        indexBase = (1:numOutputChannels:width*height*numOutputChannels)';
        index = zeros(numel(indexBase),numOutputChannels);
        for i = 1:numOutputChannels
            % Construct it as column-major index to ease later reshape
            index(:, i) = indexBase + i - 1;
        end

        % Reshape the data into a width x height x numOutputChannels matrix
        img = reshape(data(index), width, height, numOutputChannels);

        % Since reshape works column-wise, bring image back to
        % row-major order (transpose of 1st and 2nd dimension
        % Result will be a height x width x numOutputChannels image matrix
        img = permute(img, [2 1 3]);

        ave = mean(img(:, :, 1), 'all');
        
        % デバッグ用
        %{
        disp('data: ')
        disp(data(1))

        disp('mean: ')
        disp(mean(data))

        disp('len: ')
        disp(length(data))
    
        disp('R datas: ')
        disp(img(:, :, 1))
        
        disp('R mean: ')
        disp(ave)
        %}
    else
        ave = 0;
        
    end
        
end
